simulink model "part_21"  (Simulink 9.2)
settings: Solver=VariableStepAuto  StartTime=0.0  StopTime=4  RelTol=1e-3
undefined symbols (not defined in the file or in its folder): DiscIntNeverNeededParam, q0, q0_dot, Tc
settings Model: Creator=louisling  LastModifiedBy=louisling
settings DataIOCC: LimitDataPoints=off  SaveFormat=Dataset  SignalLoggingSaveFormat=Dataset  ReturnWorkspaceOutputs=on
settings OptimizationCC: LifeSpan=auto
settings DebuggingCC: UnderspecifiedInitializationDetection=Simplified  MergeDetectMultiDrivingBlocksExec=error  FcnCallInpInsideContextMsg=error  StateNameClashWarn=none  SFUnexpectedBacktrackingDiag=error  SFNoUnconditionalDefaultTransitionDiag=error  SFExecutionAtInitializationDiag=warning
settings HardwareCC: ProdBitPerPointer=64  ProdBitPerSizeT=64  ProdBitPerPtrDiffT=64  ProdLargestAtomicFloat=Float  ProdIntDivRoundTo=Zero  ProdEndianess=LittleEndian  ProdWordSize=64  ProdHWDeviceType=Intel->x86-64 (Windows64)
settings ModelReferenceCC: PropagateSignalLabelsOutOfModel=on
settings SFSimCC: SimUseLocalCustomCode=on
settings RTWCC: RTWUseLocalCustomCode=on
settings CodeAppCC: StateflowObjectComments=off
settings GRTTargetCC: TargetLangStandard=C99 (ISO)  GeneratePreprocessorConditionals=Use local settings  CombineOutputUpdateFcns=on  GRTInterface=off
settings ConfigComp: CovMetricSettings=dwe  CovHtmlReporting=off  CovSaveCumulativeToWorkspaceVar=off  CovSaveSingleToWorkspaceVar=off  CovExternalEMLEnable=on

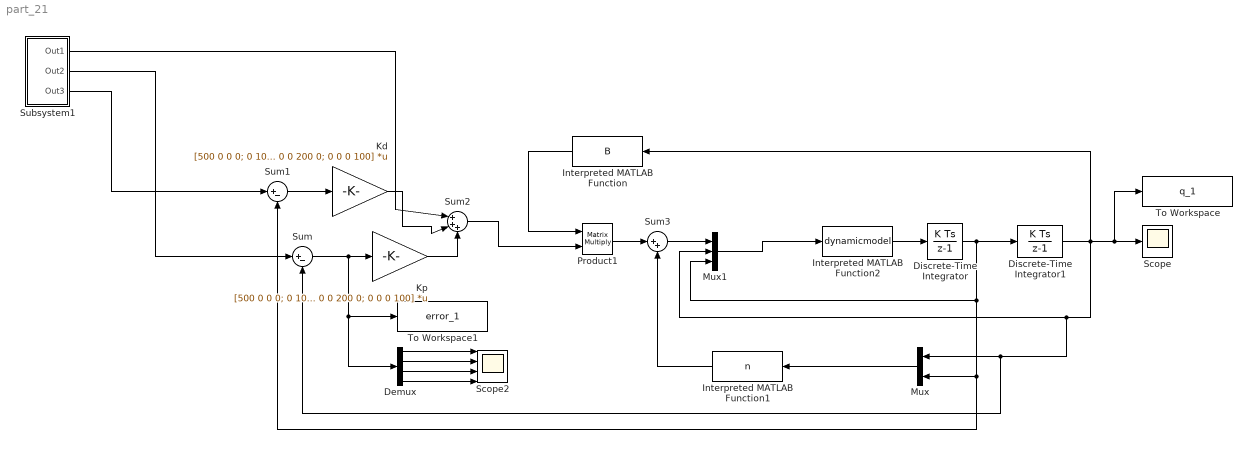
== system part_21 ==
  Demux : Demux
  Discrete-Time Integrator : DiscreteIntegrator  InitialCondition=q0_dot  SampleTime=Tc  UpperSaturationLimit=[pi/2 pi/4 1 2*pi]  ICPrevOutput=DiscIntNeverNeededParam  ICPrevScaledInput=DiscIntNeverNeededParam
  Discrete-Time Integrator1 : DiscreteIntegrator  gainval=1  InitialCondition=q0  SampleTime=Tc  LimitOutput=on  UpperSaturationLimit=[pi/2 pi/4 1 2*pi]  LowerSaturationLimit=[-pi/2 -pi/2 0.25 -2*pi]  ICPrevOutput=DiscIntNeverNeededParam  ICPrevScaledInput=DiscIntNeverNeededParam
  Interpreted MATLAB Function : MATLABFcn  MATLABFcn=B  Output1D=off
  Interpreted MATLAB Function1 : MATLABFcn  MATLABFcn=n  Output1D=off
  Interpreted MATLAB Function2 : MATLABFcn  MATLABFcn=dynamicmodel  Output1D=off
  Kd : Gain  Gain=[500 0 0 0; 0 100 0 0; 0 0 200 0; 0 0 0 100]  Multiplication=Matrix(K*u) (u vector)
  Kp : Gain  Gain=[500 0 0 0; 0 100 0 0; 0 0 200 0; 0 0 0 100]  Multiplication=Matrix(K*u) (u vector)
  Mux : Mux  Inputs=2
  Mux1 : Mux  Inputs=3
  Product1 : Product  Multiplication=Matrix(*)
  Scope : Scope
  Scope2 : Scope  NumInputPorts=4
  Subsystem1 : Subsystem
  Sum : Sum  Inputs=|+-
  Sum1 : Sum  Inputs=|+-
  Sum2 : Sum  Inputs=|+++
  Sum3 : Sum  Inputs=|++
  To Workspace : ToWorkspace  VariableName=q_1  SaveFormat=Structure With Time  SampleTime=-1
  To Workspace1 : ToWorkspace  VariableName=error_1  SaveFormat=Structure With Time  SampleTime=-1
  wires:
  Mux1/1 -> Interpreted MATLAB Function2/1
  Product1/1 -> Sum3/1
  Demux/3 -> Scope2/3
  Demux/1 -> Scope2/1
  Subsystem1/3(Out3) -> Sum1/1
  Interpreted MATLAB Function2/1 -> Discrete-Time Integrator/1
  Subsystem1/2(Out2) -> Sum/1
  Kp/1 -> Sum2/3
  Demux/4 -> Scope2/4
  Subsystem1/1(Out1) -> Sum2/1
  Discrete-Time Integrator/1 -> Discrete-Time Integrator1/1, Mux/2, Sum1/2, Mux1/3
  Kd/1 -> Sum2/2
  Demux/2 -> Scope2/2
  Interpreted MATLAB Function1/1 -> Sum3/2
  Sum/1 -> Demux/1, To Workspace1/1, Kp/1
  Sum1/1 -> Kd/1
  Sum3/1 -> Mux1/1
  Mux/1 -> Interpreted MATLAB Function1/1
  Interpreted MATLAB Function/1 -> Product1/1
  Sum2/1 -> Product1/2
  Discrete-Time Integrator1/1 -> Mux/1, Sum/2, Mux1/2, Interpreted MATLAB Function/1, To Workspace/1, Scope/1

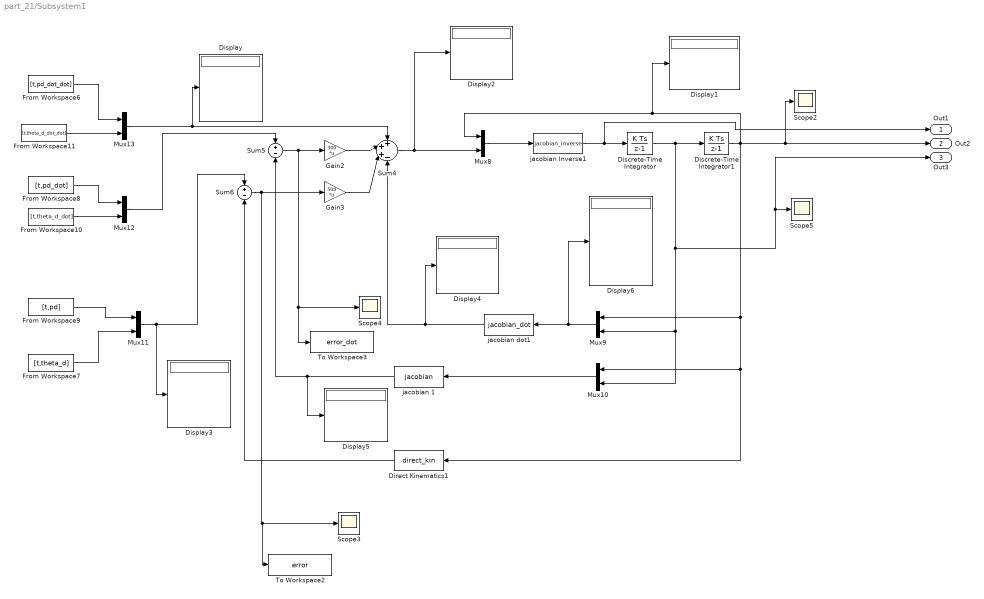
== system part_21/Subsystem1 ==
  Direct Kinematics1 : MATLABFcn  MATLABFcn=direct_kin
  Discrete-Time Integrator : DiscreteIntegrator  InitialCondition=q0_dot  SampleTime=Tc  ICPrevOutput=DiscIntNeverNeededParam  ICPrevScaledInput=DiscIntNeverNeededParam
  Discrete-Time Integrator1 : DiscreteIntegrator  InitialCondition=q0  SampleTime=Tc  ICPrevOutput=DiscIntNeverNeededParam  ICPrevScaledInput=DiscIntNeverNeededParam
  Display{,1..6} (7 alike) : Display
  From Workspace10 : FromWorkspace  VariableName=[t,theta_d_dot]  SampleTime=0
  From Workspace11 : FromWorkspace  VariableName=[t,theta_d_dot_dot]  SampleTime=0
  From Workspace6 : FromWorkspace  VariableName=[t,pd_dot_dot]  SampleTime=0
  From Workspace7 : FromWorkspace  VariableName=[t,theta_d]  SampleTime=0
  From Workspace8 : FromWorkspace  VariableName=[t,pd_dot]  SampleTime=0
  From Workspace9 : FromWorkspace  VariableName=[t,pd]  SampleTime=0
  Gain2 : Gain  Gain=300  Multiplication=Matrix(K*u)
  Gain3 : Gain  Gain=500  Multiplication=Matrix(K*u)
  Mux{8..13} (6 alike) : Mux  Inputs=2
  Scope{2..5} (4 alike) : Scope
  Sum4 : Sum  Inputs=+++-
  Sum5 : Sum  Inputs=+-
  Sum6 : Sum  Inputs=+-
  To Workspace2 : ToWorkspace  VariableName=error  SaveFormat=Structure With Time  SampleTime=-1
  To Workspace3 : ToWorkspace  VariableName=error_dot  SaveFormat=Structure With Time  SampleTime=-1
  jacobian 1 : MATLABFcn  MATLABFcn=jacobian
  jacobian Inverse1 : MATLABFcn  MATLABFcn=jacobian_inverse
  jacobian dot1 : MATLABFcn  MATLABFcn=jacobian_dot
  Out1 : Outport
  Out2 : Outport  Port=2
  Out3 : Outport  Port=3
  wires:
  Gain3/1 -> Sum4/3
  From Workspace7/1 -> Mux11/2
  jacobian 1/1 -> Display5/1, Sum5/2
  From Workspace8/1 -> Mux12/1
  From Workspace11/1 -> Mux13/2
  Discrete-Time Integrator1/1 -> Direct Kinematics1/1, Mux10/1, Mux9/1, Mux8/1, Display1/1, Out2/1, Scope2/1
  Mux10/1 -> jacobian 1/1
  Direct Kinematics1/1 -> Sum6/2
  From Workspace6/1 -> Mux13/1
  Mux8/1 -> jacobian Inverse1/1
  jacobian dot1/1 -> Display4/1, Sum4/4
  Mux13/1 -> Display/1, Sum4/1
  Sum5/1 -> To Workspace3/1, Scope4/1, Gain2/1
  From Workspace10/1 -> Mux12/2
  Gain2/1 -> Sum4/2
  Mux11/1 -> Display3/1, Sum6/1
  Sum4/1 -> Display2/1, Mux8/2
  jacobian Inverse1/1 -> Out1/1, Discrete-Time Integrator/1
  Mux9/1 -> Display6/1, jacobian dot1/1
  Discrete-Time Integrator/1 -> Mux10/2, Mux9/2, Out3/1, Scope5/1, Discrete-Time Integrator1/1
  Mux12/1 -> Sum5/1
  From Workspace9/1 -> Mux11/1
  Sum6/1 -> To Workspace2/1, Scope3/1, Gain3/1
